simulink model "simulacaoProcessoSS"  (R2018a)
settings: Solver=VariableStepAuto  StartTime=0.0  StopTime=10.0  RelTol=1e-3  EnableMultiTasking=on
values from neighbouring files (symbols this model uses):
  A = [-18.1818181818  0; 1  0]    [controltest.mat]
  B = [1 0]    [controltest.mat]
  C = [0 330]    [controltest.mat]
  K = [21.8181818182 526]    [controltest.mat]    (also in statespaceProj.m = [Ke(1) Ke(2)])
  Ki = -6.84848484848    [controltest.mat]    (also in statespaceProj.m = Ke(3))
  L = [2.69431505134 0.235812672176]    [controltest.mat]    (also in statespaceProj.m = acker(A',C',[op op2])')
settings Model: Creator=thiag  LastModifiedBy=gshimabuko
settings SolverCC: ZeroCrossAlgorithm=Adaptive
settings OptimizationCC: LifeSpan=inf
settings DebuggingCC: MaxConsecutiveZCsMsg=none  SFUnexpectedBacktrackingDiag=warning  SFNoUnconditionalDefaultTransitionDiag=warning  SFExecutionAtInitializationDiag=none
settings CodeAppCC: StateflowObjectComments=on
settings GRTTargetCC: TargetLangStandard=C89/C90 (ANSI)  GeneratePreprocessorConditionals=Disable all
settings ConfigComp: CovMetricSettings=dw  CovHtmlReporting=on  CovSaveCumulativeToWorkspaceVar=on  CovSaveSingleToWorkspaceVar=on  CovExternalEMLEnable=off

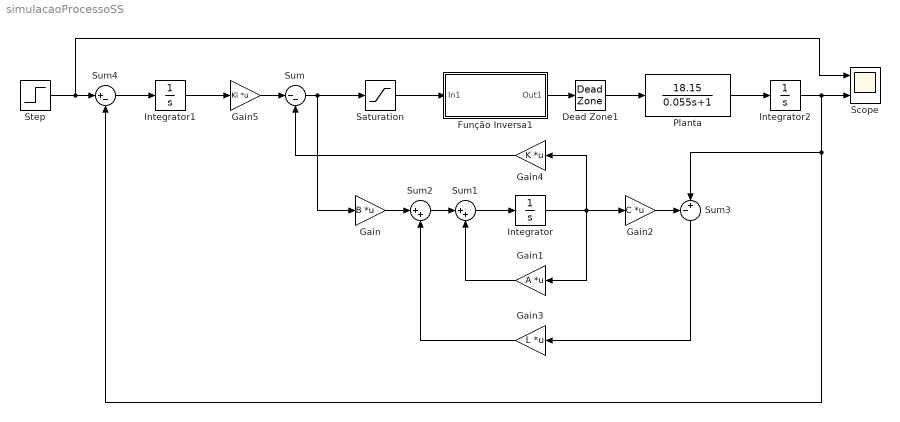
== system simulacaoProcessoSS ==
  Dead Zone1 : DeadZone  LowerValue=-0.7  UpperValue=0.95  SaturateOnIntegerOverflow=on
  Função Inversa1 : Subsystem
  Gain : Gain  Gain=B  Multiplication=Matrix(K*u)
  Gain1 : Gain  Gain=A  Multiplication=Matrix(K*u)
  Gain2 : Gain  Gain=C  Multiplication=Matrix(K*u)
  Gain3 : Gain  Gain=L  Multiplication=Matrix(K*u)
  Gain4 : Gain  Gain=K  Multiplication=Matrix(K*u)
  Gain5 : Gain  Gain=Ki  Multiplication=Matrix(K*u)
  Integrator : Integrator
  Integrator1 : Integrator
  Integrator2 : Integrator
  Planta : TransferFcn  Numerator=[18.15]  Denominator=[0.055 1]
  Saturation : Saturate  UpperLimit=10  LowerLimit=-10
  Scope : Scope  NumInputPorts=2
  Step : Step  After=45  SampleTime=0
  Sum : Sum  Inputs=|--
  Sum1 : Sum  Inputs=|++
  Sum2 : Sum  Inputs=|++
  Sum3 : Sum  Inputs=-+|
  Sum4 : Sum  Inputs=|+-
  wires:
  Sum/1 -> Saturation/1, Gain/1
  Sum1/1 -> Integrator/1
  Integrator/1 -> Gain4/1, Gain1/1, Gain2/1
  Gain1/1 -> Sum1/2
  Gain/1 -> Sum2/1
  Sum2/1 -> Sum1/1
  Gain2/1 -> Sum3/1
  Gain4/1 -> Sum/2
  Step/1 -> Sum4/1, Scope/1
  Gain5/1 -> Sum/1
  Sum3/1 -> Gain3/1
  Sum4/1 -> Integrator1/1
  Integrator1/1 -> Gain5/1
  Gain3/1 -> Sum2/2
  Dead Zone1/1 -> Planta/1
  Planta/1 -> Integrator2/1
  Integrator2/1 -> Sum4/2, Sum3/2, Scope/2
  Função Inversa1/1(Out1) -> Dead Zone1/1
  Saturation/1 -> Função Inversa1/1(In1)

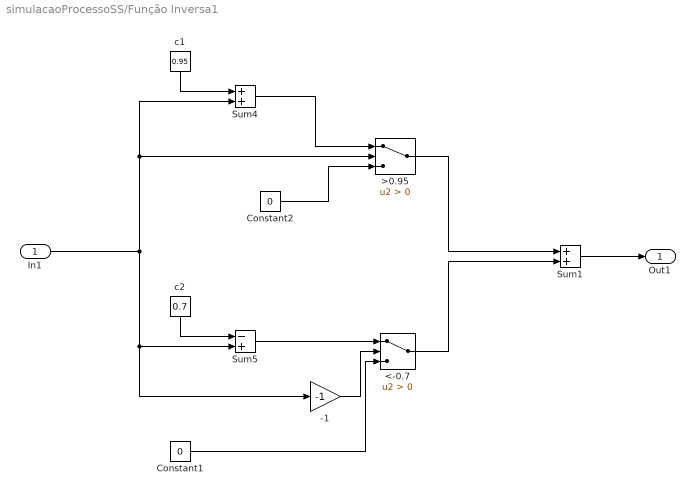
== system simulacaoProcessoSS/Função Inversa1 ==
  In1 : Inport
  -1 : Gain  Gain=-1
  "<-0.7 " : Switch  Criteria=u2 > Threshold
  ">0.95 " : Switch  Criteria=u2 > Threshold
  Constant1 : Constant  Value=0
  Constant2 : Constant  Value=0
  Sum1 : Sum
  Sum4 : Sum
  Sum5 : Sum  Inputs=-+
  c1 : Constant  Value=0.95
  c2 : Constant  Value=0.7
  Out1 : Outport
  wires:
  c2/1 -> Sum5/1
  In1/1 -> Sum4/2, ">0.95 "/2, -1/1, Sum5/2
  -1/1 -> "<-0.7 "/2
  Sum5/1 -> "<-0.7 "/1
  Constant1/1 -> "<-0.7 "/3
  "<-0.7 "/1 -> Sum1/2
  ">0.95 "/1 -> Sum1/1
  Sum1/1 -> Out1/1
  c1/1 -> Sum4/1
  Sum4/1 -> ">0.95 "/1
  Constant2/1 -> ">0.95 "/3
